simulink model "SecRwLtStLgrstInwdOtwdHolderChk"  (R2018b)
settings: Solver=FixedStepDiscrete  StartTime=0.0  StopTime=10.0  FixedStep=0.01  RelTol=1e-3
libraries: simulink x2
settings Model: Creator=sn2xws  LastModifiedBy=sn2xws
settings Model: ModifiedHistory=|
  | 2023/11/7Bug 555794 童锁需要停止 21-26
  | 25.7.7 V3.13.0 新增Md61 Md62
settings DataIOCC: SaveFormat=StructureWithTime
settings OptimizationCC: DefaultParameterBehavior=Inlined  EnhancedBackFolding=on  PassReuseOutputArgsAs=Individual arguments  ZeroExternalMemoryAtStartup=off  ZeroInternalMemoryAtStartup=off  OptimizeBlockOrder=speed  DifferentSizesBufferReuse=on  OptimizationCustomize=off
settings DebuggingCC: ParameterTunabilityLossMsg=error
settings ModelReferenceCC: ModelReferenceNumInstancesAllowed=Single
settings SFSimCC: MATLABDynamicMemAlloc=off
settings RTWCC: SystemTargetFile=autosar.tlc  GenCodeOnly=on  TemplateMakefile=ert_default_tmf  Description=AUTOSAR  GenerateReport=on  IncludeHyperlinkInReport=on  LaunchReport=on  GenerateTraceInfo=on  GenerateTraceReport=on  GenerateTraceReportSl=on  GenerateTraceReportSf=on  GenerateTraceReportEml=on
settings CodeAppCC: ForceParamTrailComments=on  IgnoreCustomStorageClasses=off  OperatorAnnotations=on  SimulinkDataObjDesc=on  SFDataObjDesc=on  InsertBlockDesc=on
settings STFCustomTargetCC: TargetLangStandard=C99 (ISO)  MultiwordLength=256  ParMdlRefBuildCompliant=on  CompOptLevelCompliant=on  IncludeMdlTerminateFcn=off  CombineOutputUpdateFcns=on  SuppressErrorStatus=on  ERTCustomFileBanners=on  SupportNonFinite=off  SupportComplex=off  SupportContinuousTime=off  SupportNonInlinedSFcns=off  RemoveResetFunc=on  MATLABClassNameForMDSCustomization=Simulink.SoftwareTarget.ERTCustomization  AutosarCompliant=on  UseToolchainInfoCompliant=on  LookupTableObjectStructAxisOrder=2,1,3,4,...  LUTObjectStructOrderEvenSpacing=Size,Table,Breakpoints  SystemTargetFile=autosar.tlc
settings ERTTargetCC: TargetLangStandard=C99 (ISO)  ConcurrentExecutionCompliant=off  IncludeMdlTerminateFcn=off  SuppressErrorStatus=on  SupportNonFinite=off  SupportComplex=off  ModelStepFunctionPrototypeControlCompliant=off  CPPClassGenCompliant=off  AutosarCompliant=on  LookupTableObjectStructAxisOrder=2,1,3,4,...  LUTObjectStructOrderEvenSpacing=Size,Table,Breakpoints  InlinedParameterPlacement=NonHierarchical  ERTCustomFileTemplate=example_file_process.tlc  ERTFilePackagingFormat=Compact

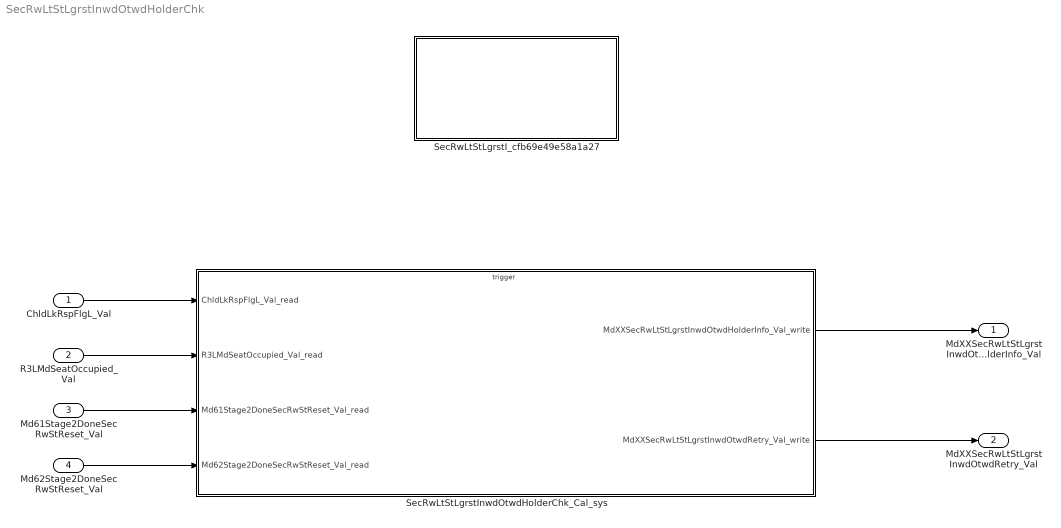
== system SecRwLtStLgrstInwdOtwdHolderChk ==
  ChldLkRspFlgL_Val : Inport  OutDataTypeStr=boolean  PortDimensions=1
  R3LMdSeatOccupied_Val : Inport  Port=2  OutDataTypeStr=boolean  PortDimensions=1
  Md61Stage2DoneSecRwStReset_Val : Inport  Port=3  OutDataTypeStr=boolean  PortDimensions=1
  Md62Stage2DoneSecRwStReset_Val : Inport  Port=4  OutDataTypeStr=boolean  PortDimensions=1
  SecRwLtStLgrstI_cfb69e49e58a1a27 : Subsystem
  SecRwLtStLgrstInwdOtwdHolderChk_Cal_sys : Subsystem
  MdXXSecRwLtStLgrstInwdOtwdHolderInfo_Val : Outport  OutDataTypeStr=uint32  PortDimensions=1
  MdXXSecRwLtStLgrstInwdOtwdRetry_Val : Outport  Port=2  OutDataTypeStr=uint32  PortDimensions=1
  wires:
  ChldLkRspFlgL_Val/1 -> SecRwLtStLgrstInwdOtwdHolderChk_Cal_sys/1(ChldLkRspFlgL_Val_read)
  R3LMdSeatOccupied_Val/1 -> SecRwLtStLgrstInwdOtwdHolderChk_Cal_sys/2(R3LMdSeatOccupied_Val_read)
  SecRwLtStLgrstInwdOtwdHolderChk_Cal_sys/1(MdXXSecRwLtStLgrstInwdOtwdHolderInfo_Val_write) -> MdXXSecRwLtStLgrstInwdOtwdHolderInfo_Val/1
  Md61Stage2DoneSecRwStReset_Val/1 -> SecRwLtStLgrstInwdOtwdHolderChk_Cal_sys/3(Md61Stage2DoneSecRwStReset_Val_read)
  Md62Stage2DoneSecRwStReset_Val/1 -> SecRwLtStLgrstInwdOtwdHolderChk_Cal_sys/4(Md62Stage2DoneSecRwStReset_Val_read)
  SecRwLtStLgrstInwdOtwdHolderChk_Cal_sys/2(MdXXSecRwLtStLgrstInwdOtwdRetry_Val_write) -> MdXXSecRwLtStLgrstInwdOtwdRetry_Val/1

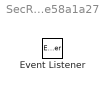
== system SecRwLtStLgrstInwdOtwdHolderChk/SecRwLtStLgrstI_cfb69e49e58a1a27 ==
  Event Listener : EventListener  EventName=reset

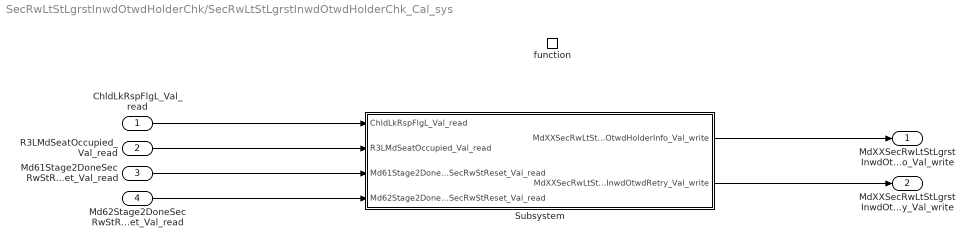
== system SecRwLtStLgrstInwdOtwdHolderChk/SecRwLtStLgrstInwdOtwdHolderChk_Cal_sys ==
  ChldLkRspFlgL_Val_read : Inport
  R3LMdSeatOccupied_Val_read : Inport  Port=2
  Md61Stage2DoneSecRwStReset_Val_read : Inport  Port=3
  Md62Stage2DoneSecRwStReset_Val_read : Inport  Port=4
  function : TriggerPort  TriggerType=function-call  IsSimulinkFunction=on  FunctionName=SecRwLtStLgrstInwdOtwdHolderChk_Cal  VariantControl=(inherit)
  Subsystem : Subsystem
  MdXXSecRwLtStLgrstInwdOtwdHolderInfo_Val_write : Outport
      settings: EnsureOutportIsVirtual=on
  MdXXSecRwLtStLgrstInwdOtwdRetry_Val_write : Outport  Port=2
      settings: EnsureOutportIsVirtual=on
  wires:
  Subsystem/1(MdXXSecRwLtStLgrstInwdOtwdHolderInfo_Val_write) -> MdXXSecRwLtStLgrstInwdOtwdHolderInfo_Val_write/1
  R3LMdSeatOccupied_Val_read/1 -> Subsystem/2(R3LMdSeatOccupied_Val_read)
  ChldLkRspFlgL_Val_read/1 -> Subsystem/1(ChldLkRspFlgL_Val_read)
  Subsystem/2(MdXXSecRwLtStLgrstInwdOtwdRetry_Val_write) -> MdXXSecRwLtStLgrstInwdOtwdRetry_Val_write/1
  Md62Stage2DoneSecRwStReset_Val_read/1 -> Subsystem/4(Md62Stage2DoneSecRwStReset_Val_read)
  Md61Stage2DoneSecRwStReset_Val_read/1 -> Subsystem/3(Md61Stage2DoneSecRwStReset_Val_read)

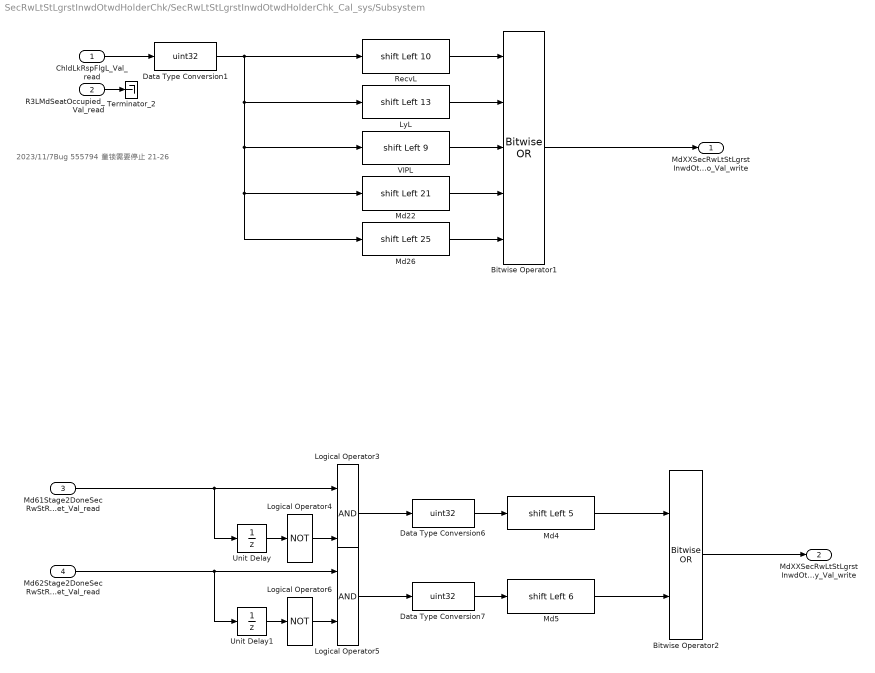
== system SecRwLtStLgrstInwdOtwdHolderChk/SecRwLtStLgrstInwdOtwdHolderChk_Cal_sys/Subsystem ==
  note: 2023/11/7Bug 555794 童锁需要停止 21-26
  ChldLkRspFlgL_Val_read : Inport
  R3LMdSeatOccupied_Val_read : Inport  Port=2
  Md61Stage2DoneSecRwStReset_Val_read : Inport  Port=3
  Md62Stage2DoneSecRwStReset_Val_read : Inport  Port=4
  Bitwise Operator1 : simulink/Logic and Bit Operations/Bitwise Operator  logicop=OR  UseBitMask=off  NumInputPorts=5  BitMask=bin2dec('11011001')  BitMaskRealWorld=Stored Integer
  Bitwise Operator2 : simulink/Logic and Bit Operations/Bitwise Operator  logicop=OR  UseBitMask=off  NumInputPorts=2  BitMask=bin2dec('11011001')  BitMaskRealWorld=Stored Integer
  Data Type Conversion1 : DataTypeConversion  OutDataTypeStr=uint32
  Data Type Conversion6 : DataTypeConversion  OutDataTypeStr=uint32
  Data Type Conversion7 : DataTypeConversion  OutDataTypeStr=uint32
  Logical Operator3 : Logic  AllPortsSameDT=off  OutDataTypeStr=boolean
  Logical Operator4 : Logic  Operator=NOT  AllPortsSameDT=off  OutDataTypeStr=boolean
  Logical Operator5 : Logic  AllPortsSameDT=off  OutDataTypeStr=boolean
  Logical Operator6 : Logic  Operator=NOT  AllPortsSameDT=off  OutDataTypeStr=boolean
  LyL : ArithShift  BitShiftNumber=13  BitShiftDirection=Left
  Md22 : ArithShift  BitShiftNumber=21  BitShiftDirection=Left
  Md26 : ArithShift  BitShiftNumber=25  BitShiftDirection=Left
  Md4 : ArithShift  BitShiftNumber=5  BitShiftDirection=Left
  Md5 : ArithShift  BitShiftNumber=6  BitShiftDirection=Left
  RecvL : ArithShift  BitShiftNumber=10  BitShiftDirection=Left
  Terminator_2 : Terminator
  Unit Delay : UnitDelay  SampleTime=-1
  Unit Delay1 : UnitDelay  SampleTime=-1
  VIPL : ArithShift  BitShiftNumber=9  BitShiftDirection=Left
  MdXXSecRwLtStLgrstInwdOtwdHolderInfo_Val_write : Outport
      settings: EnsureOutportIsVirtual=on
  MdXXSecRwLtStLgrstInwdOtwdRetry_Val_write : Outport  Port=2
      settings: EnsureOutportIsVirtual=on
  wires:
  ChldLkRspFlgL_Val_read/1 -> Data Type Conversion1/1
  Bitwise Operator1/1 -> MdXXSecRwLtStLgrstInwdOtwdHolderInfo_Val_write/1
  R3LMdSeatOccupied_Val_read/1 -> Terminator_2/1
  VIPL/1 -> Bitwise Operator1/3
  Data Type Conversion1/1 -> RecvL/1, Md26/1, Md22/1, VIPL/1, LyL/1
  LyL/1 -> Bitwise Operator1/2
  RecvL/1 -> Bitwise Operator1/1
  Md22/1 -> Bitwise Operator1/4
  Md26/1 -> Bitwise Operator1/5
  Bitwise Operator2/1 -> MdXXSecRwLtStLgrstInwdOtwdRetry_Val_write/1
  Md61Stage2DoneSecRwStReset_Val_read/1 -> Logical Operator3/1, Unit Delay/1
  Md4/1 -> Bitwise Operator2/1
  Unit Delay1/1 -> Logical Operator6/1
  Logical Operator3/1 -> Data Type Conversion6/1
  Logical Operator4/1 -> Logical Operator3/2
  Md5/1 -> Bitwise Operator2/2
  Data Type Conversion6/1 -> Md4/1
  Logical Operator6/1 -> Logical Operator5/2
  Unit Delay/1 -> Logical Operator4/1
  Md62Stage2DoneSecRwStReset_Val_read/1 -> Logical Operator5/1, Unit Delay1/1
  Data Type Conversion7/1 -> Md5/1
  Logical Operator5/1 -> Data Type Conversion7/1
